simulink model "power_V2Gtest"  (R2015a)
settings: Solver=ode45  StartTime=0.0  StopTime=0.0001  RelTol=1e-3
undefined symbols (not defined in the file or in its folder): A, B, C, data, Dd, j
undefined symbols (not defined in the file): to, V2G
libraries: powerlib x22, sps_avr x1, V2Glib x1, powerlib_meascontrol x1
settings Model: Creator=Srinivas Baskar  LastModifiedBy=Harish

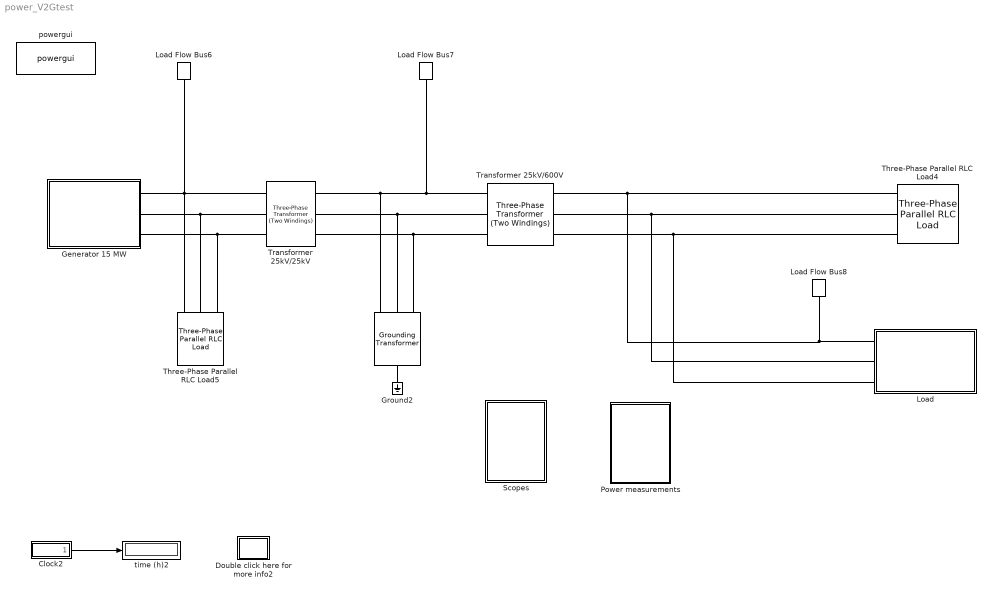
== system power_V2Gtest ==
  " " : powerlib/Elements/Grounding Transformer   UNITS=pu  NominalPower="[10e6   60]"  NominalVoltage=25e3  ZeroSequenceImpedance_pu=[0.00083333 9.4248]  MagnetizationBranch_pu=[5000 6283.2]  ZeroSequenceImpedance_SI=[0.25 7.5]  MagnetizationBranch_SI=[31250 31250]  Measurements=None
  Clock2 : Subsystem
  Double click here for more info2 : Subsystem
      settings: OpenFcn=showdemo(bdroot(gcb))
      mask Display: disp('?')
  Generator 15 MW : Subsystem
  Ground2 : powerlib/Elements/Ground  LConnTagsString=a
  "Load " : Subsystem
  Load Flow Bus6 : powerlib/Measurements/Load Flow Bus  LConnTagsString=a  ID=BUS_1  Vbase=25e3  Vref=1  Vangle=0  VLF=1  angleLF=0
      settings: AttributesFormatString=%<ID>\n%<Vbase>V\n%<VLF>pu\n%<angleLF>deg.
  Load Flow Bus7 : powerlib/Measurements/Load Flow Bus  LConnTagsString=a  ID=BUS_2  Vbase=25e3  Vref=1  Vangle=0  VLF=0.9783  angleLF=-0.1322
      settings: AttributesFormatString=%<ID>\n%<Vbase>V\n%<VLF>pu\n%<angleLF>deg.
  Load Flow Bus8 : powerlib/Measurements/Load Flow Bus  LConnTagsString=a  ID=BUS_3  Vbase=1e3  Vref=1  Vangle=0  VLF=0.9583  angleLF=-3.174
      settings: AttributesFormatString=%<ID>\n%<Vbase>V\n%<VLF>pu\n%<angleLF>deg.
  Power measurements : Subsystem
  Scopes : Subsystem
  Three-Phase Parallel RLC Load4 : powerlib/Elements/Three-Phase Parallel RLC Load  LConnTagsString=A|B|C  Configuration=Y (grounded)  NominalVoltage=(1000)*0.958281  NominalFrequency=60  ActivePower=1e3  InductivePower=0  CapacitivePower=0  Measurements=None  LoadType=constant PQ
  Three-Phase Parallel RLC Load5 : powerlib/Elements/Three-Phase Parallel RLC Load  LConnTagsString=A|B|C  Configuration=Y (grounded)  NominalVoltage=(25000)*1  NominalFrequency=60  ActivePower=1e3  InductivePower=0  CapacitivePower=0  Measurements=None  LoadType=constant PQ
  Transformer 25kV/25kV : powerlib/Elements/Three-Phase Transformer (Two Windings)  Winding1Connection=Yg  Winding2Connection=Yg  CoreType=Three single-phase transformers  SetSaturation=off  Hysteresis=off  DataFile='hysteresis'  SetInitialFlux=off  Measurements=None  UNITS=pu  NominalPower=[ 20e6 , 60 ]  Winding1=[25e3 , 0.002 , 0.08 ]  Winding2=[ 25e3 , 0.002 , 0.08 ]  Rm=500  Lm=500  L0=0.5  Saturation=[ 0,0 ; 0.0024,1.2 ; 1.0,1.52 ]  InitialFluxes=[ 0.8 , -0.8 , 0.7 ]  MoreParameters=off  BreakLoop=off  DataType=off  TransfoNumber=1
  Transformer 25kV/600V : powerlib/Elements/Three-Phase Transformer (Two Windings)  Winding1Connection=Yg  Winding2Connection=Yg  CoreType=Three single-phase transformers  SetSaturation=off  Hysteresis=off  DataFile='hysteresis'  SetInitialFlux=off  Measurements=None  UNITS=pu  NominalPower=[ 20e6 , 60 ]  Winding1=[25e3 , 0.002 , 0.08 ]  Winding2=[ 600 , 0.002 , 0.08 ]  Rm=500  Lm=500  L0=0.5  Saturation=[ 0,0 ; 0.0024,1.2 ; 1.0,1.52 ]  InitialFluxes=[ 0.8 , -0.8 , 0.7 ]  MoreParameters=off  BreakLoop=off  DataType=off  TransfoNumber=1
  powergui : powerlib/powergui  Priority=1  SimulationMode=Phasor  SolverType=Tustin  SampleTime=50e-6  frequency=60  SPID=off  DisableSnubberDevices=off  DisableRonSwitches=off  DisableVfSwitches=off  SwTol=0  DisplayEquations=off  Interpol=off  methode=off  Ts=100  FunctionMessages=off  echomessages=off  HookPort=off  EnableUseOfTLC=off  x0status=blocks  frequencyindice=60  Pbase=10e6  ErrMax=0.0001  Iterations=50  UnitsV=kV  UnitsW=MW  buscounter=0  RestoreLinks=warning  ResistiveCurrentMeasurement=off  Frange=[0:2:500]  Ylog=off  Xlog=on  ShowGrid=off  save=off  variable=ZData  structure=0  ZoomFFT=off  StartTime=0.0  cycles=1  DisplayStyle=1  fundamental=60  FreqAxis=off  MaxFrequency=1000  frequencyindicesteady=1  RmsSteady=1  display=off
  time (h)2 : Display
      settings: Format=bank
  wires:
  Clock2/1(" ") -> time (h)2/1
  connections:
  "Load "/LConn3 -- Three-Phase Parallel RLC Load4/LConn3 -- Transformer 25kV/600V/RConn3
  Transformer 25kV/25kV/RConn3 -- Transformer 25kV/600V/LConn3 -- " "/LConn3
  Three-Phase Parallel RLC Load5/LConn1 -- Load Flow Bus6/LConn1 -- Transformer 25kV/25kV/LConn1 -- Generator 15 MW/RConn1
  "Load "/LConn1 -- Three-Phase Parallel RLC Load4/LConn1 -- Transformer 25kV/600V/RConn1 -- Load Flow Bus8/LConn1
  "Load "/LConn2 -- Three-Phase Parallel RLC Load4/LConn2 -- Transformer 25kV/600V/RConn2
  Transformer 25kV/25kV/RConn2 -- Transformer 25kV/600V/LConn2 -- " "/LConn2
  Three-Phase Parallel RLC Load5/LConn3 -- Transformer 25kV/25kV/LConn3 -- Generator 15 MW/RConn3
  Three-Phase Parallel RLC Load5/LConn2 -- Transformer 25kV/25kV/LConn2 -- Generator 15 MW/RConn2
  " "/RConn1 -- Ground2/LConn1
  Transformer 25kV/25kV/RConn1 -- Load Flow Bus7/LConn1 -- Transformer 25kV/600V/LConn1 -- " "/LConn1

== system power_V2Gtest/Clock2 ==
  Clock : Clock
  Gain : Gain  Gain=1/3600
  " " : Outport
  wires:
  Gain/1 -> " "/1
  Clock/1 -> Gain/1

== system power_V2Gtest/Double click here for more info2 ==

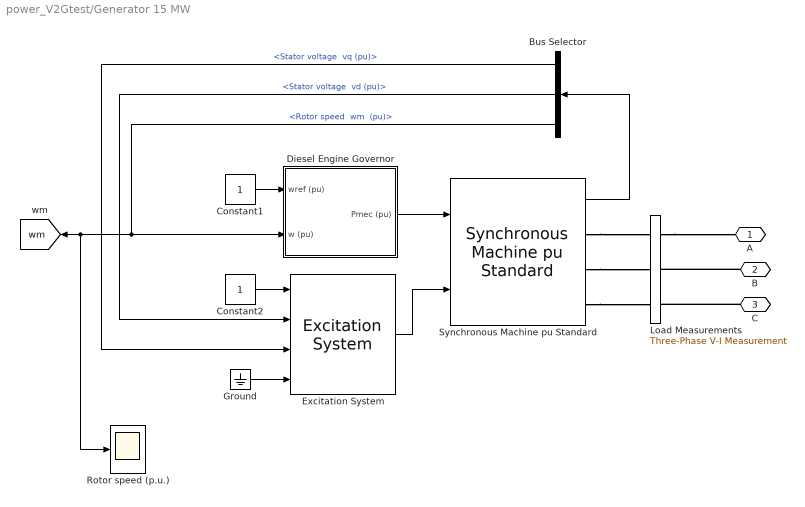
== system power_V2Gtest/Generator 15 MW ==
  " Load Measurements" : powerlib/Measurements/Three-Phase V-I Measurement  VoltageMeasurement=phase-to-ground  SetLabelV=on  LabelV=Vabc1  Vpu=off  VpuLL=off  CurrentMeasurement=yes  SetLabelI=on  LabelI=Iabc1  Ipu=off  Pbase=2*1.5e6/0.9  Vbase=25e3  OutputType=Complex  PhasorSimulation=on  PSBequivalent=0
  Bus Selector : BusSelector  OutputSignals="dq0 components.Stator voltage  vq (pu),dq0 components.Stator voltage  vd (pu),Mechanical.Rotor speed  wm  (pu)"
  Constant1 : Constant
  Constant2 : Constant
  Diesel Engine Governor : Subsystem  mask(Diesel Engine & Governor){K=29, Tr=[0.01 0.02 0.2], Ta=[0.25 0.009 0.0384], Tlim=[0 1.1], Td=0.024, Pm0=0.1361}
      mask prompts: K "Regulator gain K:"; Tr "Regulator time constants [T1 T2 T3 ] (s) :"; Ta "Actuator time constants [T4 T5 T6] (s) :"; Tlim "Torque limits [Tmin Tmax] (pu) :"; Td "Engine time delay Td (s) :"; Pm0 "Initial value of mechanical power  Pm0 (pu) :"
      mask help:
      | This block implements a diesel engine and governor system:
      | 1st and 2nd inputs: Desired and actual speed (pu)
      | Output: Diesel engine mechanical power.Motor inertia should be combined with generator.
      | Controller transfer function:
      |      Hc=K.(1+T3.s)/(1+T1.s+T1.T2.s^2)
      | Actuator transfer function :
      |      Ha= (1+T4.s) / [ (s (1+T5.s)(1+T6.s) ]
      | Motor :
      |      Time delay Td
      |
      | (See reference in Tutorial Session 5)
  Excitation System : sps_avr/Excitation System  tr=20e-3  reg=[ 300, 0.001 ]  exc=[ 1, 0 ]  tgr=[ 0, 0 ]  damp=[ 0.001, 0.1 ]  sat=[ 0, 0 ]  lim=[ -11.5, 11.5, 0 ]  v0=[1 1.2473]
  Ground : Ground
  Rotor speed (p.u.) : Scope
      settings: TimeRange=86400  YMin=0.9955  YMax=1.005  SaveName=wm1
  Synchronous Machine pu Standard : powerlib/Machines/Synchronous Machine pu Standard  PresetModel=No  MechanicalLoad=Mechanical power Pm  ShowDetailedParameters=on  RotorType=Salient-pole  Units=per unit standard parameters  MeasurementBus=off  NominalParameters="[ 15E6  25e3   60]"  Reactances1=[ 1.81, 0.3, 0.23, 1.76, 0.65, 0.25, 0.15 ]  Reactances2="[ 1.305, 0.296, 0.252, 0.474,  0.243,  0.18 ]"  dAxisTimeConstants=Open-circuit  qAxisTimeConstants=Short-circuit  TimeConstants1="[ 4.4849  0.0681  0.1  ]"  TimeConstants2=[ 8.0, 0.03, 1.0, 0.07 ]  TimeConstants3="[  4.49  0.0681  0.0513  ]"  TimeConstants4=[ 8.0, 0.03, 0.3371, 0.0295 ]  TimeConstants5=[ 1.01, 0.053, 0.1 ]  TimeConstants6=[ 1.3201, 0.023, 1.0, 0.07 ]  TimeConstants7=[0.012 0.003 0.003]  TimeConstants8=[ 1.3201, 0.0231, 0.3371, 0.0295 ]  StatorResistance=0.003  Mechanical=[3.7 0 1 ]  PolePairs=20  InitialConditions=[0 -86.6365 0.2279 0.2279 0.2279 -53.3785 -173.379 66.6215 1.24735]  SetSaturation=off  Saturation=[0.6404,0.7127,0.8441,0.9214,0.9956,1.082,1.19,1.316,1.457;0.7,0.7698,0.8872,0.9466,0.9969,1.046,1.1,1.151,1.201]  LoadFlowParameters=[1,0,0,0,0]  TsPowergui=0  TsBlock=-1  IterativeModel=Trapezoidal non iterative  BusType=swing  Pref=0  Qref=0  Qmin=-inf  Qmax=inf  PLF=0  QLF=0
  A : PMIOPort  Port=1  Side=Right
  B : PMIOPort  Port=2  Side=Right
  C : PMIOPort  Port=3  Side=Right
  tag scope: wm=global
  wires:
  Bus Selector/3 -> Diesel Engine Governor/2(w (pu)), Rotor speed (p.u.)/1, [wm]  "<Rotor speed  wm  (pu)>"
  Constant1/1 -> Diesel Engine Governor/1(wref (pu))
  Diesel Engine Governor/1(Pmec (pu)) -> Synchronous Machine pu Standard/1
  Excitation System/1 -> Synchronous Machine pu Standard/2
  Constant2/1 -> Excitation System/1
  Bus Selector/2 -> Excitation System/2  "<Stator voltage  vd (pu)>"
  Bus Selector/1 -> Excitation System/3  "<Stator voltage  vq (pu)>"
  Synchronous Machine pu Standard/1 -> Bus Selector/1
  Ground/1 -> Excitation System/4
  connections:
  " Load Measurements"/RConn1 -- A/RConn1
  C/RConn1 -- " Load Measurements"/RConn3
  B/RConn1 -- " Load Measurements"/RConn2
  Synchronous Machine pu Standard/RConn3 -- " Load Measurements"/LConn3
  Synchronous Machine pu Standard/RConn2 -- " Load Measurements"/LConn2
  Synchronous Machine pu Standard/RConn1 -- " Load Measurements"/LConn1

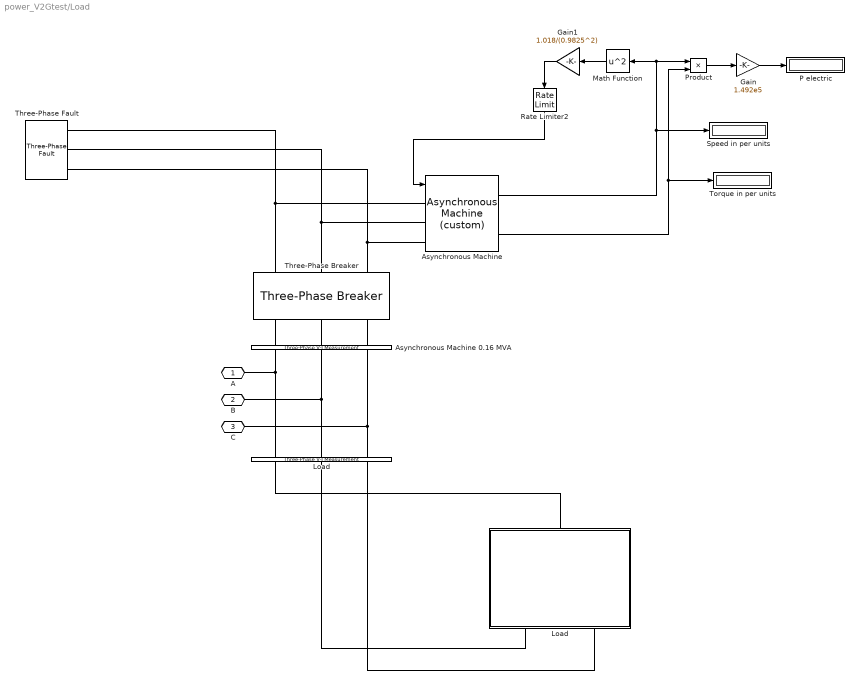
== system power_V2Gtest/Load  ==
  " Asynchronous Machine 0.16 MVA " : powerlib/Measurements/Three-Phase V-I Measurement  VoltageMeasurement=phase-to-ground  SetLabelV=on  LabelV=Vasm  Vpu=off  VpuLL=off  CurrentMeasurement=yes  SetLabelI=on  LabelI=Iasm  Ipu=off  Pbase=2*1.5e6/0.9  Vbase=25e3  OutputType=Complex  PhasorSimulation=on  PSBequivalent=0
  " Load " : powerlib/Measurements/Three-Phase V-I Measurement  VoltageMeasurement=phase-to-ground  SetLabelV=on  LabelV=Vload  Vpu=off  VpuLL=off  CurrentMeasurement=yes  SetLabelI=on  LabelI=Iload  Ipu=off  Pbase=2*1.5e6/0.9  Vbase=25e3  OutputType=Complex  PhasorSimulation=on  PSBequivalent=0
  "Asynchronous Machine " : V2Glib/Asynchronous Machine (custom)  RotorType=Squirrel-cage  PresetModel=No  MechanicalLoad=Torque Tm  ShowDetailedParameters=on  ReferenceFrame=Rotor  Units=pu  MeasurementBus=on  NominalParameters=[1.5e+05 600 60]  Stator=[0.01117 0.04832]  Rotor=[0.006 0.04832]  Cage1=[0.01909 0.0397]  Cage2=[0.01909 0.0397]  Lm=2.424  Mechanical=[0.3096 0.01511 2]  PolePairs=2  InitialConditions=[1 0 0 0 0 0 0 0]  SimulateSaturation=off  Saturation="[0.212,0.4201,0.8125,1.0979,1.4799,2.2457,3.2586,4.5763,6.4763 ;   0.5,0.7,0.9,1,1.1,1.2 ,1.3,1.4,1.5]"  LoadFlowParameters=0  TsPowergui=0  TsBlock=-1  IterativeModel=Trapezoidal non iterative  Pmec=2e6
  Gain : Gain  Gain=1.492e5
  Gain1 : Gain  Gain=1.018/(0.9825^2)
  "Load " : Subsystem  mask{nomPower=10, PF=0.95, timestep=60, datas=V2G.CONSUMPTION}
      mask prompts: nomPower "Nominal Power (MW)"; PF "Power factor"; timestep "Timestep (minutes)"; datas "Consumption datas"
      mask DialogControl DescGroupVar Prompt: Load profile
      mask DialogControl DescTextVar Prompt: The load profile allows you to fix a nominal power and and a power factor. It is also needed to specify the timestep used for the consumption datas. Finally, a vector expresses the consumption profile. It has to be expressed in per unit. It is imperative that the length of the vector fits with the timestep used.
  Math Function : Math  Operator=square  SaturateOnIntegerOverflow=on
  P electric : Display
  Product : Product
  Rate Limiter2 : RateLimiter  RisingSlewLimit=1e4  FallingSlewLimit=-1e4  SampleTimeMode=inherited
  "Speed in per units " : Display
  Three-Phase Breaker : powerlib/Elements/Three-Phase Breaker  InitialState=open  SwitchA=on  SwitchB=on  SwitchC=on  SwitchTimes=[ 3*3600]  External=off  BreakerResistance=0.001  SnubberResistance=1e6  SnubberCapacitance=inf  Measurements=None
  Three-Phase Fault : powerlib/Elements/Three-Phase Fault  InitialStates=0  FaultA=off  FaultB=off  FaultC=off  GroundFault=on  SwitchTimes=[4*3600 4*3600+100]  External=off  SwitchStatus=NaN  FaultResistance=0.001  GroundResistance=0.01  SnubberResistance=1e6  SnubberCapacitance=inf  Measurements=None
  Torque in per units : Display
  A : PMIOPort  Port=1  Side=Left
  B : PMIOPort  Port=2  Side=Left
  C : PMIOPort  Port=3  Side=Left
  wires:
  Gain1/1 -> Rate Limiter2/1
  "Asynchronous Machine "/1 -> "Speed in per units "/1, Product/1, Math Function/1
  "Asynchronous Machine "/2 -> Product/2, Torque in per units/1
  Product/1 -> Gain/1
  Gain/1 -> P electric/1
  Math Function/1 -> Gain1/1
  Rate Limiter2/1 -> "Asynchronous Machine "/1
  connections:
  " Asynchronous Machine 0.16 MVA "/RConn2 -- B/RConn1 -- " Load "/RConn2
  " Asynchronous Machine 0.16 MVA "/RConn3 -- " Load "/RConn3 -- C/RConn1
  " Load "/RConn1 -- A/RConn1 -- " Asynchronous Machine 0.16 MVA "/RConn1
  "Asynchronous Machine "/LConn2 -- Three-Phase Fault/LConn2 -- Three-Phase Breaker/LConn2
  Three-Phase Fault/LConn3 -- "Asynchronous Machine "/LConn3 -- Three-Phase Breaker/LConn3
  Three-Phase Breaker/RConn1 -- " Asynchronous Machine 0.16 MVA "/LConn1
  Three-Phase Breaker/RConn2 -- " Asynchronous Machine 0.16 MVA "/LConn2
  Three-Phase Breaker/RConn3 -- " Asynchronous Machine 0.16 MVA "/LConn3
  Three-Phase Fault/LConn1 -- "Asynchronous Machine "/LConn1 -- Three-Phase Breaker/LConn1
  " Load "/LConn1 -- "Load "/RConn1
  " Load "/LConn2 -- "Load "/LConn1
  " Load "/LConn3 -- "Load "/LConn2

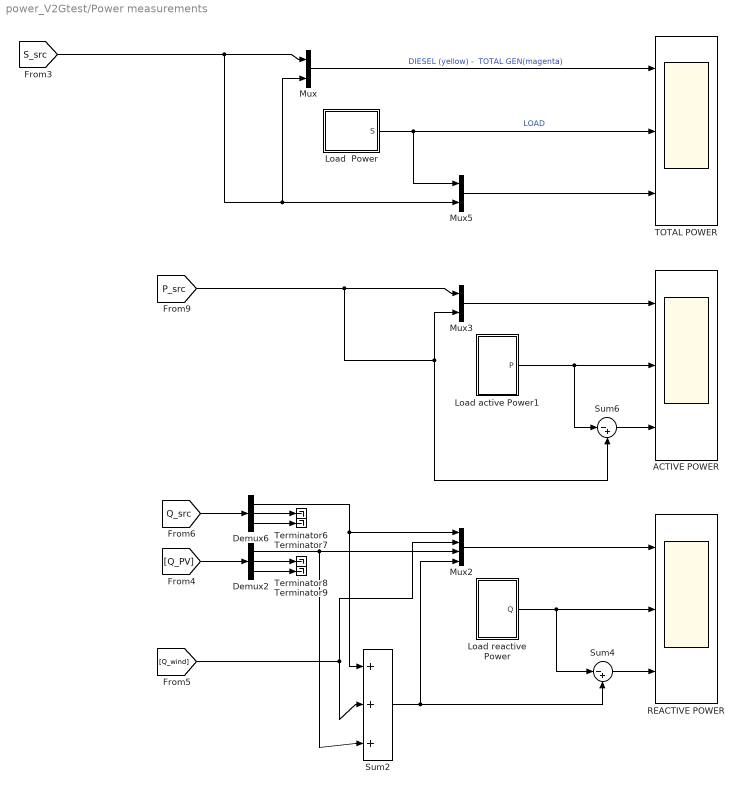
== system power_V2Gtest/Power measurements ==
  ACTIVE POWER : Scope  NumInputPorts=3
      settings: TimeRange=86394.68034477012  YMin=-1127645.502645526~0~0  YMax=14321145.12471653~14000000~194678.5071649832  SaveName=ScopeData9  Decimation=20
  Demux2 : Demux  Outputs=3
  Demux6 : Demux  Outputs=3
  Load  Power : Subsystem
  Load active Power1 : Subsystem
  Load reactive Power : Subsystem
  Mux : Mux  Inputs=2
  Mux2 : Mux
  Mux3 : Mux  Inputs=2
  Mux5 : Mux  Inputs=2
  REACTIVE POWER : Scope  NumInputPorts=3
      settings: TimeRange=86394.68034477012  YMin=-639880.9523809515~29417.73813057679~0  YMax=7141203.703703707~4200987.36115234~2993413.800705456  SaveName=ScopeData7  Decimation=20
  Sum2 : Sum  Inputs=|+++
  Sum4 : Sum  Inputs=|-+
  Sum6 : Sum  Inputs=|-+
  TOTAL POWER : Scope  NumInputPorts=3
      settings: TimeRange=86395.43113750442  YMin=0~0~123381.0870346278  YMax=16020911.12187349~14000000~16409684.57560659  SaveName=ScopeData5  Decimation=20
  Terminator{6..9} (4 alike) : Terminator
  wires:
  [Q_src] -> Demux6/1
  [S_src] -> Mux/2, Mux5/2, Mux/1
  Demux6/1 -> Sum2/1, Mux2/1
  [Q_wind] -> Mux2/2, Sum2/2
  Sum2/1 -> Sum4/2, Mux2/4
  Mux/1 -> TOTAL POWER/1  "DIESEL (yellow) -  TOTAL GEN(magenta)"
  Mux2/1 -> REACTIVE POWER/1
  Sum4/1 -> REACTIVE POWER/3
  Mux5/1 -> TOTAL POWER/3
  Load  Power/1(S) -> TOTAL POWER/2, Mux5/1  "LOAD"
  [Q_PV] -> Demux2/1
  Demux2/1 -> Sum2/3, Mux2/3
  Load reactive Power/1("Q ") -> Sum4/1, REACTIVE POWER/2
  [P_src] -> Mux3/2, Sum6/2, Mux3/1
  Mux3/1 -> ACTIVE POWER/1
  Load active Power1/1(P) -> Sum6/1, ACTIVE POWER/2
  Sum6/1 -> ACTIVE POWER/3
  Demux6/2 -> Terminator6/1
  Demux6/3 -> Terminator7/1
  Demux2/2 -> Terminator8/1
  Demux2/3 -> Terminator9/1

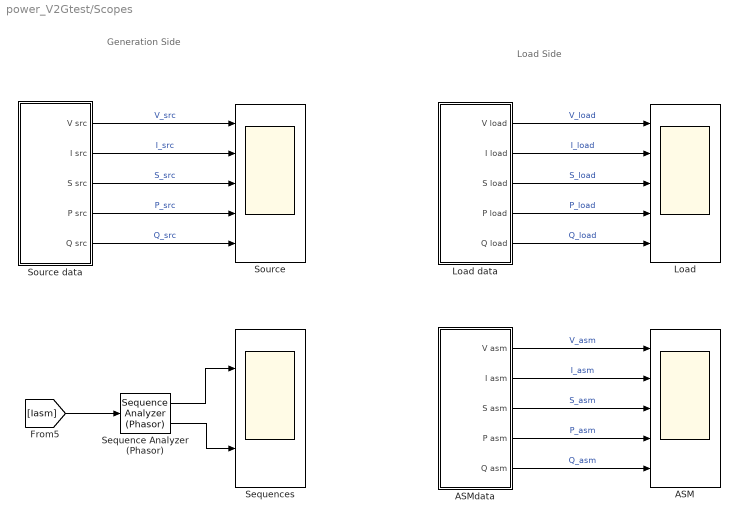
== system power_V2Gtest/Scopes ==
  note: Generation
      | Side
  note: Load Side
  ASM : Scope  NumInputPorts=5
      settings: TimeRange=86394.68034477012  YMin=383.346641994195~0~0~-279310.3448275863~-231272.2948870416  YMax=518.2077387266461~464.9227110582633~270214.030915576~0~92152.19976218522  SaveName=ScopeData10  Decimation=20
  ASMdata : Subsystem
  Load : Scope  NumInputPorts=5
      settings: TimeRange=86394.68034477012  YMin=395.7726844069046~6091.95402298851~4224137.931034483~-11810344.8275862~-4000000  YMax=499.0979539956536~18045.97701149426~12500000~-3706896.551724136~-655172.4137931094  Decimation=20
  "Load data " : Subsystem
  Sequence Analyzer (Phasor) : powerlib_meascontrol/Measurements/Sequence Analyzer (Phasor)  seq=Positive Negative Zero
  Sequences : Scope  NumInputPorts=2
      settings: TimeRange=86394.68034477012  YMin=0~-200  YMax=3500~200  SaveName=ScopeData6  Decimation=20
  Source : Scope  NumInputPorts=5
      settings: TimeRange=86394.68034477012  YMin=19667.0693040594~0~0~0~0  YMax=20918.20386543416~400~14997637.78661004~12955761.02158985~8413549.565165743  SaveName=ScopeData2  Decimation=20
  Source data : Subsystem
  wires:
  Source data/5(Q src) -> Source/5  "Q_src"
  Source data/4(P src) -> Source/4  "P_src"
  Source data/3(S src) -> Source/3  "S_src"
  Source data/2(I src) -> Source/2  "I_src"
  Source data/1(V src) -> Source/1  "V_src"
  "Load data "/5(Q load) -> Load/5  "Q_load"
  "Load data "/1(V load) -> Load/1  "V_load"
  "Load data "/2(I load) -> Load/2  "I_load"
  "Load data "/3(S load) -> Load/3  "S_load"
  "Load data "/4(P load) -> Load/4  "P_load"
  ASMdata/5(Q asm) -> ASM/5  "Q_asm"
  ASMdata/1(V asm) -> ASM/1  "V_asm"
  ASMdata/2(I asm) -> ASM/2  "I_asm"
  ASMdata/3(S asm) -> ASM/3  "S_asm"
  ASMdata/4(P asm) -> ASM/4  "P_asm"
  Sequence Analyzer (Phasor)/1 -> Sequences/1
  Sequence Analyzer (Phasor)/2 -> Sequences/2
  [Iasm] -> Sequence Analyzer (Phasor)/1

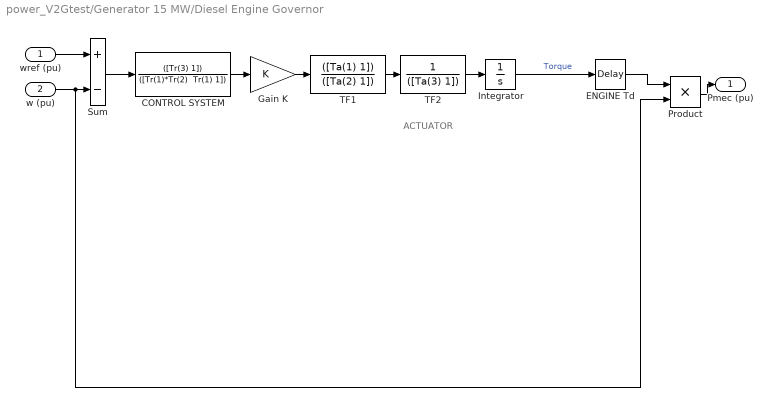
== system power_V2Gtest/Generator 15 MW/Diesel Engine Governor ==
  note: ACTUATOR
  wref (pu) : Inport
  w (pu) : Inport  Port=2
  CONTROL SYSTEM : TransferFcn  Numerator=([Tr(3) 1])  Denominator="([Tr(1)*Tr(2)  Tr(1) 1])"
  ENGINE Td : TransportDelay  DelayTime=Td  InitialOutput=Pm0
  Gain K : Gain  Gain=K  SaturateOnIntegerOverflow=on  OutDataTypeStr=Inherit: Same as input  ParamDataTypeStr=Inherit: Same as input
  Integrator : Integrator  InitialCondition=Pm0  LimitOutput=on  UpperSaturationLimit=Tlim(2)  LowerSaturationLimit=Tlim(1)
  Product : Product  SaturateOnIntegerOverflow=on  InputSameDT=on  OutDataTypeStr=Inherit: Same as first input
  Sum : Sum  Inputs=+-  SaturateOnIntegerOverflow=on  InputSameDT=on  OutDataTypeStr=Inherit: Same as first input
  TF1 : TransferFcn  Numerator=([Ta(1) 1])  Denominator=([Ta(2) 1])
  TF2 : TransferFcn  Numerator=1  Denominator=([Ta(3) 1])
  Pmec (pu) : Outport  InitialOutput=0
  wires:
  Gain K/1 -> TF1/1
  Sum/1 -> CONTROL SYSTEM/1
  CONTROL SYSTEM/1 -> Gain K/1
  TF1/1 -> TF2/1
  w (pu)/1 -> Product/2, Sum/2
  ENGINE Td/1 -> Product/1
  wref (pu)/1 -> Sum/1
  Product/1 -> Pmec (pu)/1
  TF2/1 -> Integrator/1
  Integrator/1 -> ENGINE Td/1  "Torque"

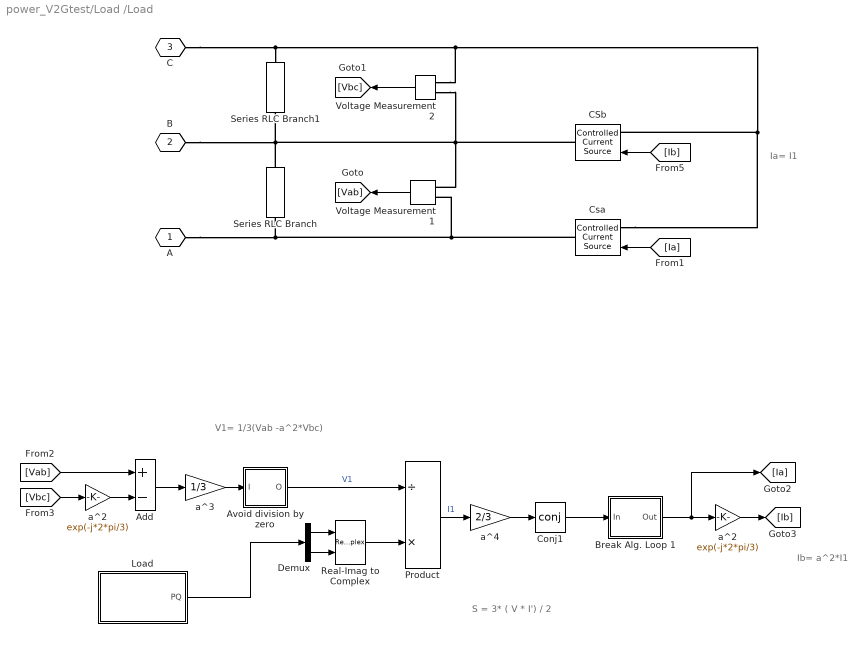
== system power_V2Gtest/Load /Load  ==
  note: Ia= I1
  note: V1= 1/3(Vab -a^2*Vbc)
  note: S = 3* ( V * I') / 2
  note: Ib= a^2*I1
  Add : Sum  Inputs=+-
  Avoid division by zero : Subsystem
  Break Alg. Loop 1 : Subsystem
  CSb : powerlib/Electrical Sources/Controlled Current Source  Initialize=on  Source_Type=AC  Amplitude=9355.5  Phase=(2.751-2*pi/3)*180/pi  Frequency=60  Measurements=Current
  Conj1 : Math  Operator=conj  SaturateOnIntegerOverflow=on
  Csa : powerlib/Electrical Sources/Controlled Current Source  Initialize=on  Source_Type=AC  Amplitude=9355.5  Phase=2.751*180/pi  Frequency=60  Measurements=Current
  Demux : Demux  Outputs=2
  Load : Subsystem
  Product : Product  Inputs=/*  SaturateOnIntegerOverflow=on  InputSameDT=on  OutDataTypeStr=Inherit: Same as first input
  Real-Imag to Complex : RealImagToComplex
  Series RLC Branch : powerlib/Elements/Series RLC Branch  LConnTagsString=__new0  RConnTagsString=__new0  BranchType=R  Resistance=1e6  Inductance=1e-3  SetiL0=off  InitialCurrent=0  Capacitance=1e-6  Setx0=off  InitialVoltage=0  Measurements=None
  Series RLC Branch1 : powerlib/Elements/Series RLC Branch  LConnTagsString=__new0  RConnTagsString=__new0  BranchType=R  Resistance=1e6  Inductance=1e-3  SetiL0=off  InitialCurrent=0  Capacitance=1e-6  Setx0=off  InitialVoltage=0  Measurements=None
  Voltage Measurement1 : powerlib/Measurements/Voltage Measurement  PhasorSimulation=on  OutputType=Complex  PSBequivalent=0
  Voltage Measurement2 : powerlib/Measurements/Voltage Measurement  PhasorSimulation=on  OutputType=Complex  PSBequivalent=0
  a^2 : Gain  Gain=exp(-j*2*pi/3)  SaturateOnIntegerOverflow=on  OutDataTypeStr=Inherit: Same as input  ParamDataTypeStr=Inherit: Same as input
  "a^2 " : Gain  Gain=exp(-j*2*pi/3)  SaturateOnIntegerOverflow=on  OutDataTypeStr=Inherit: Same as input  ParamDataTypeStr=Inherit: Same as input
  a^3 : Gain  Gain=1/3  SaturateOnIntegerOverflow=on  OutDataTypeStr=Inherit: Same as input  ParamDataTypeStr=Inherit: Same as input
  a^4 : Gain  Gain=2/3  SaturateOnIntegerOverflow=on  OutDataTypeStr=Inherit: Same as input  ParamDataTypeStr=Inherit: Same as input
  A : PMIOPort  Tag=PMCPort  Port=1  Side=Right
  B : PMIOPort  Tag=PMCPort  Port=2  Side=Left
  C : PMIOPort  Tag=PMCPort  Port=3  Side=Left
  wires:
  Real-Imag to Complex/1 -> Product/2
  Product/1 -> a^4/1  "I1"
  a^2/1 -> [Ib]
  a^3/1 -> Avoid division by zero/1(I)
  Add/1 -> a^3/1
  [Vab] -> Add/1
  [Vbc] -> "a^2 "/1
  "a^2 "/1 -> Add/2
  a^4/1 -> Conj1/1
  Demux/1 -> Real-Imag to Complex/1
  Demux/2 -> Real-Imag to Complex/2
  Load/1(PQ) -> Demux/1
  Avoid division by zero/1(O) -> Product/1  "V1"
  Conj1/1 -> Break Alg. Loop 1/1(In)
  Break Alg. Loop 1/1(Out) -> [Ia], a^2/1
  [Ib] -> CSb/1
  [Ia] -> Csa/1
  Voltage Measurement1/1 -> [Vab]
  Voltage Measurement2/1 -> [Vbc]
  connections:
  B/RConn1 -- Voltage Measurement2/LConn1 -- Voltage Measurement1/LConn2 -- CSb/RConn1 -- Series RLC Branch/RConn1 -- Series RLC Branch1/LConn1
  C/RConn1 -- Csa/LConn1 -- CSb/LConn1 -- Voltage Measurement2/LConn2 -- Series RLC Branch1/RConn1
  A/RConn1 -- Voltage Measurement1/LConn1 -- Csa/RConn1 -- Series RLC Branch/LConn1

== system power_V2Gtest/Power measurements/Load  Power ==
  Sum : Sum  Inputs=++++
  S : Outport
  wires:
  Sum/1 -> S/1
  [S_EV] -> Sum/2
  [S_charg] -> Sum/3
  [S_load] -> Sum/1
  [S_asm] -> Sum/4

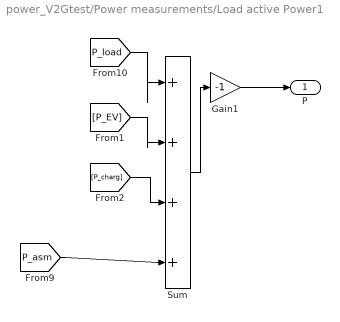
== system power_V2Gtest/Power measurements/Load active Power1 ==
  Gain1 : Gain  Gain=-1
  Sum : Sum  Inputs=|++++
  P : Outport
  wires:
  [P_asm] -> Sum/4
  Sum/1 -> Gain1/1
  [P_charg] -> Sum/3
  [P_load] -> Sum/1
  [P_EV] -> Sum/2
  Gain1/1 -> P/1

== system power_V2Gtest/Power measurements/Load reactive Power ==
  Gain1 : Gain  Gain=-1
  Sum : Sum  Inputs=|++++
  "Q " : Outport
  wires:
  Sum/1 -> Gain1/1
  [Q_charg] -> Sum/3
  [Q_load] -> Sum/1
  [Q_EV] -> Sum/2
  Gain1/1 -> "Q "/1
  [Q_asm] -> Sum/4

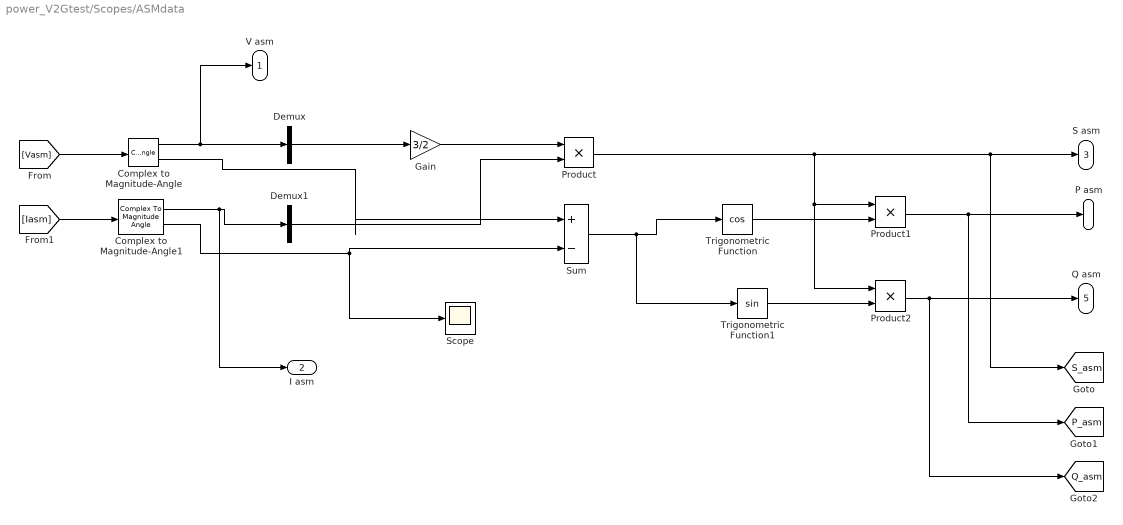
== system power_V2Gtest/Scopes/ASMdata ==
  Complex to Magnitude-Angle : ComplexToMagnitudeAngle
  Complex to Magnitude-Angle1 : ComplexToMagnitudeAngle
  Demux : Demux  Outputs=1
  Demux1 : Demux  Outputs=1
  Gain : Gain  Gain=3/2
  Product : Product
  Product1 : Product
  Product2 : Product
  Scope : Scope
      settings: SaveName=ScopeData3
  Sum : Sum  Inputs=|+-
  Trigonometric Function : Trigonometry  Operator=cos
  Trigonometric Function1 : Trigonometry
  V asm : Outport
  I asm : Outport  Port=2
  S asm : Outport  Port=3
  P asm : Outport  Port=4
  Q asm : Outport  Port=5
  tag scope: P_asm=global, Q_asm=global, S_asm=global
  wires:
  Product2/1 -> Q asm/1, [Q_asm]
  Product1/1 -> P asm/1, [P_asm]
  Trigonometric Function/1 -> Product1/2
  Trigonometric Function1/1 -> Product2/2
  Sum/1 -> Trigonometric Function/1, Trigonometric Function1/1
  Complex to Magnitude-Angle/2 -> Sum/1
  [Iasm] -> Complex to Magnitude-Angle1/1
  [Vasm] -> Complex to Magnitude-Angle/1
  Complex to Magnitude-Angle1/2 -> Sum/2, Scope/1
  Product/1 -> Product1/1, Product2/1, S asm/1, [S_asm]
  Demux1/1 -> Product/2
  Gain/1 -> Product/1
  Complex to Magnitude-Angle1/1 -> Demux1/1, I asm/1
  Complex to Magnitude-Angle/1 -> Demux/1, V asm/1
  Demux/1 -> Gain/1

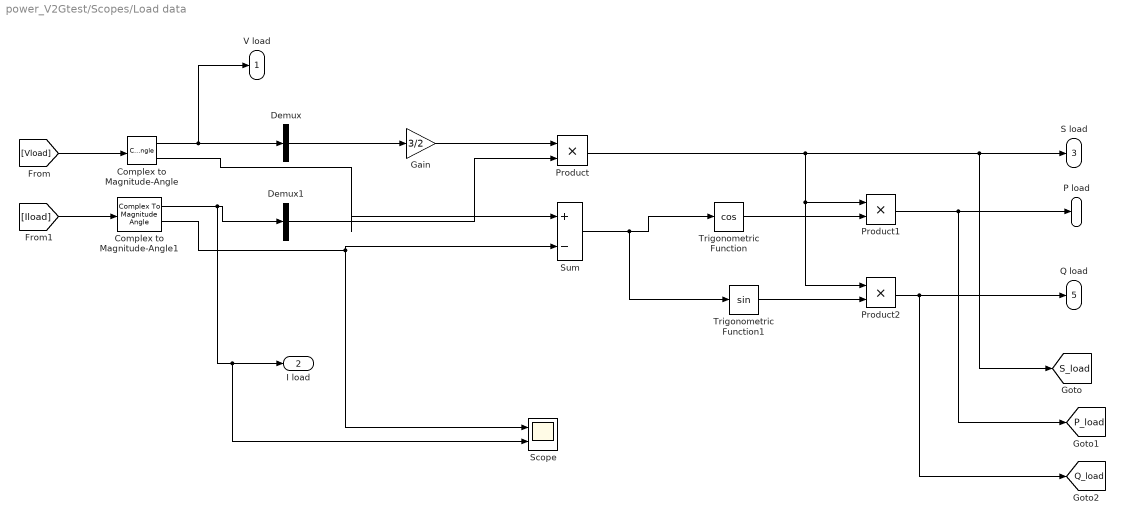
== system power_V2Gtest/Scopes/Load data  ==
  Complex to Magnitude-Angle : ComplexToMagnitudeAngle
  Complex to Magnitude-Angle1 : ComplexToMagnitudeAngle
  Demux : Demux  Outputs=1
  Demux1 : Demux  Outputs=1
  Gain : Gain  Gain=3/2
  Product : Product
  Product1 : Product
  Product2 : Product
  Scope : Scope  NumInputPorts=2
      settings: YMin=-3.5~0  YMax=3.5~10000  SaveName=ScopeData3
  Sum : Sum  Inputs=|+-
  Trigonometric Function : Trigonometry  Operator=cos
  Trigonometric Function1 : Trigonometry
  V load : Outport
  I load : Outport  Port=2
  S load : Outport  Port=3
  P load : Outport  Port=4
  Q load : Outport  Port=5
  tag scope: P_load=global, Q_load=global, S_load=global
  wires:
  Demux/1 -> Gain/1
  Complex to Magnitude-Angle/1 -> V load/1, Demux/1
  Complex to Magnitude-Angle1/1 -> Scope/2, I load/1, Demux1/1
  Gain/1 -> Product/1
  Demux1/1 -> Product/2
  Product/1 -> [S_load], S load/1, Product2/1, Product1/1
  Complex to Magnitude-Angle1/2 -> Scope/1, Sum/2
  [Vload] -> Complex to Magnitude-Angle/1
  [Iload] -> Complex to Magnitude-Angle1/1
  Complex to Magnitude-Angle/2 -> Sum/1
  Sum/1 -> Trigonometric Function1/1, Trigonometric Function/1
  Trigonometric Function1/1 -> Product2/2
  Trigonometric Function/1 -> Product1/2
  Product1/1 -> [P_load], P load/1
  Product2/1 -> [Q_load], Q load/1

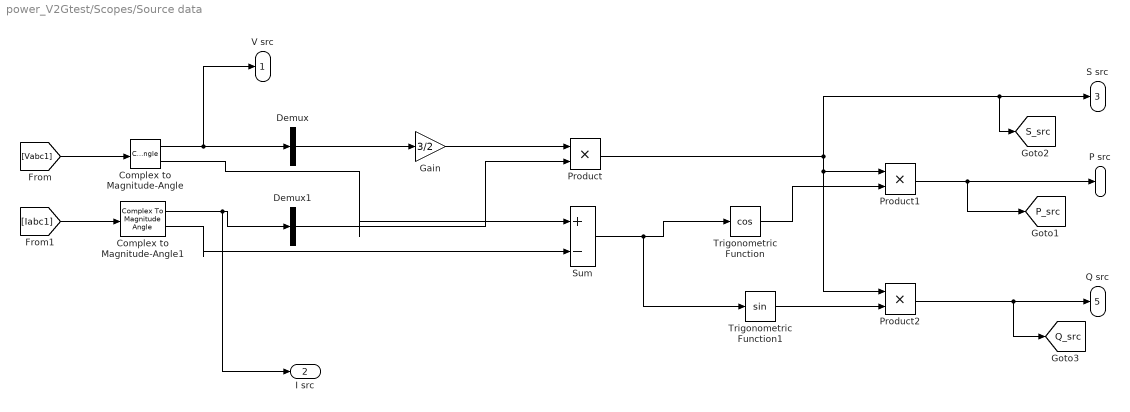
== system power_V2Gtest/Scopes/Source data ==
  Complex to Magnitude-Angle : ComplexToMagnitudeAngle
  Complex to Magnitude-Angle1 : ComplexToMagnitudeAngle
  Demux : Demux  Outputs=1
  Demux1 : Demux  Outputs=1
  Gain : Gain  Gain=3/2
  Product : Product
  Product1 : Product
  Product2 : Product
  Sum : Sum  Inputs=|+-
  Trigonometric Function : Trigonometry  Operator=cos
  Trigonometric Function1 : Trigonometry
  V src : Outport
  I src : Outport  Port=2
  S src : Outport  Port=3
  P src : Outport  Port=4
  Q src : Outport  Port=5
  tag scope: P_src=global, Q_src=global, S_src=global
  wires:
  Product2/1 -> [Q_src], Q src/1
  Product1/1 -> P src/1, [P_src]
  Trigonometric Function/1 -> Product1/2
  Trigonometric Function1/1 -> Product2/2
  Sum/1 -> Trigonometric Function/1, Trigonometric Function1/1
  Complex to Magnitude-Angle/2 -> Sum/1
  [Iabc1] -> Complex to Magnitude-Angle1/1
  [Vabc1] -> Complex to Magnitude-Angle/1
  Complex to Magnitude-Angle1/2 -> Sum/2
  Product/1 -> Product1/1, Product2/1, S src/1, [S_src]
  Demux1/1 -> Product/2
  Gain/1 -> Product/1
  Complex to Magnitude-Angle1/1 -> Demux1/1, I src/1
  Complex to Magnitude-Angle/1 -> Demux/1, V src/1
  Demux/1 -> Gain/1

== system power_V2Gtest/Load /Load /Avoid division by zero ==
  I : Inport
  Complex to Magnitude-Angle : ComplexToMagnitudeAngle
  Magnitude-Angle to Complex : MagnitudeAngleToComplex
  Saturation1 : Saturate  UpperLimit=inf  LowerLimit=1e-6
  O : Outport
  wires:
  I/1 -> Complex to Magnitude-Angle/1
  Saturation1/1 -> Magnitude-Angle to Complex/1
  Complex to Magnitude-Angle/1 -> Saturation1/1
  Magnitude-Angle to Complex/1 -> O/1
  Complex to Magnitude-Angle/2 -> Magnitude-Angle to Complex/2

== system power_V2Gtest/Load /Load /Break Alg. Loop 1 ==
  In : Inport
  Complex to Real-Imag : ComplexToRealImag
  Real-Imag to Complex : RealImagToComplex
  imag : Subsystem  mask(Transfer Function with Initial Outputs){N=[1], D=[to  1], Y0=0, U0=0}
      mask prompts: N "Numerator:"; D "Denominator:"; Y0 "Initial output:"; U0 "Initial input:"
      mask help: Vector expressions for numerator, and denominator. Coefficients are in descending powers of s.
      mask init:
      | [A,B,C,Dd]=tf2ss(N,D);if (isempty(Y0));[m,n]=size(A);X0=zeros(1,m); end; if (isempty(U0));[m,p]=size(B);U0=zeros(1,p);end;X0=getxo(A,B,C,Dd,U0,Y0,0);
      mask Help: Specify the initial output for the transfer function.  An optimization routine attempts to determine the appropriate initial states so that the specified initial output is achieved.  For more details, see the m-file getxo.m
      mask Display: dpoly(N,D,'s')
  real : Subsystem  mask(Transfer Function with Initial Outputs){N=[1], D=[to 1], Y0=0, U0=0}
      mask prompts: N "Numerator:"; D "Denominator:"; Y0 "Initial output:"; U0 "Initial input:"
      mask help: Vector expressions for numerator, and denominator. Coefficients are in descending powers of s.
      mask init:
      | [A,B,C,Dd]=tf2ss(N,D);if (isempty(Y0));[m,n]=size(A);X0=zeros(1,m); end; if (isempty(U0));[m,p]=size(B);U0=zeros(1,p);end;X0=getxo(A,B,C,Dd,U0,Y0,0);
      mask Help: Specify the initial output for the transfer function.  An optimization routine attempts to determine the appropriate initial states so that the specified initial output is achieved.  For more details, see the m-file getxo.m
      mask Display: dpoly(N,D,'s')
  Out : Outport
  wires:
  Complex to Real-Imag/1 -> real/1(In1)
  Complex to Real-Imag/2 -> imag/1(In1)
  In/1 -> Complex to Real-Imag/1
  Real-Imag to Complex/1 -> Out/1
  real/1(Out1) -> Real-Imag to Complex/1
  imag/1(Out1) -> Real-Imag to Complex/2

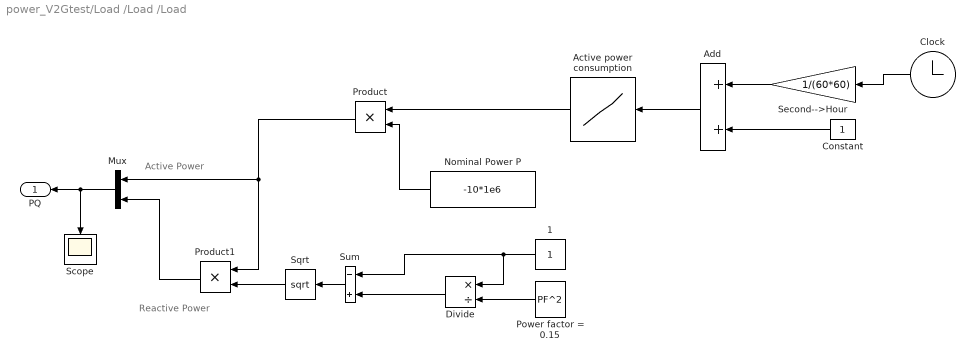
== system power_V2Gtest/Load /Load /Load ==
  note: Reactive Power
  note: Active Power
  " Active power consumption " : Lookup_n-D  NumberOfTableDimensions=1  BreakpointsForDimension1=[1:timestep/60:8760]  BeginIndexSearchUsingPreviousIndexResult=on  Table=data  InternalRulePriority=Speed  RndMeth=Simplest  InputSameDT=on
  1 : Constant
  Add : Sum
  Clock : Clock
  Constant : Constant
  Divide : Product  Inputs=*/
  Mux : Mux  Inputs=2
  Nominal Power P : Constant  Value=-10*1e6
  Power factor = 0.15 : Constant  Value=PF^2
  Product : Product
  Product1 : Product
  Scope : Scope
      settings: YMin=-6e+06  YMax=-1.75e+06  SaveName=ScopeData4  Decimation=20
  Second-->Hour : Gain  Gain=1/(60*60)
  Sqrt : Sqrt  SaturateOnIntegerOverflow=on
  Sum : Sum  Inputs=-+
  PQ : Outport
  wires:
  Constant/1 -> Add/2
  1/1 -> Sum/1, Divide/1
  Second-->Hour/1 -> Add/1
  Sum/1 -> Sqrt/1
  Power factor = 0.15/1 -> Divide/2
  Add/1 -> " Active power consumption "/1
  Nominal Power P/1 -> Product/2
  Clock/1 -> Second-->Hour/1
  Sqrt/1 -> Product1/2
  Product/1 -> Product1/1, Mux/1
  Divide/1 -> Sum/2
  " Active power consumption "/1 -> Product/1
  Mux/1 -> Scope/1, PQ/1
  Product1/1 -> Mux/2

== system power_V2Gtest/Load /Load /Break Alg. Loop 1/imag ==
  In1 : Inport
  State Space : StateSpace  A=A  B=B  C=C  D=Dd  X0=X0
  Out1 : Outport  InitialOutput=0
  wires:
  State Space/1 -> Out1/1
  In1/1 -> State Space/1

== system power_V2Gtest/Load /Load /Break Alg. Loop 1/real ==
  In1 : Inport
  State Space : StateSpace  A=A  B=B  C=C  D=Dd  X0=X0
  Out1 : Outport  InitialOutput=0
  wires:
  State Space/1 -> Out1/1
  In1/1 -> State Space/1
